simulink model "tutorial3"  (R2023b)
settings: Solver=FixedStepAuto  StartTime=0.0  StopTime=10.0  FixedStep=1e-3  RelTol=1e-3  EnableMultiTasking=on
libraries: frdmk64flib x5, etargetslib x2
settings Model: ExtModeTrigDuration=5  Creator=user  LastModifiedBy=user
settings OptimizationCC: EnhancedBackFolding=on  PassReuseOutputArgsAs=Individual arguments  ZeroExternalMemoryAtStartup=off  ZeroInternalMemoryAtStartup=off  MaxStackSize=64  OptimizeBlockOrder=speed  DifferentSizesBufferReuse=on  OptimizationCustomize=off  EfficientTunableParamExpr=on
settings DebuggingCC: ParameterTunabilityLossMsg=error
settings HardwareCC: ProdBitPerPointer=32  ProdBitPerSizeT=32  ProdBitPerPtrDiffT=32  ProdLargestAtomicInteger=Long  ProdLargestAtomicFloat=Double  ProdWordSize=32  ProdHWDeviceType=ARM Compatible->ARM Cortex
settings SFSimCC: MATLABDynamicMemAlloc=off
settings RTWCC: Description=Embedded Coder  SystemTargetFile=ert.tlc  HardwareBoard=NXP FRDM-K64F  TLCOptions="-aInlineSetEventsForThisBaseRateFcn=TLC_FALSE -aSuppressMultiTaskScheduler=TLC_FALSE  -aRateBasedStepFcn=0"  TemplateMakefile=ert_default_tmf  Toolchain=GNU Tools for ARM Embedded Processors
settings CodeAppCC: ForceParamTrailComments=on  IgnoreCustomStorageClasses=off  OperatorAnnotations=on  SimulinkDataObjDesc=on  SFDataObjDesc=on  InsertBlockDesc=on
settings ERTTargetCC: ExtModeTransport=4  ExtModeMexFile=sendToCommService

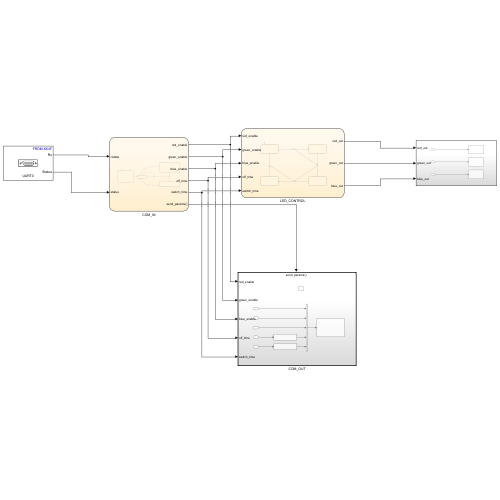
[thumbnail: Simulink's stored preview of the top-level diagram]
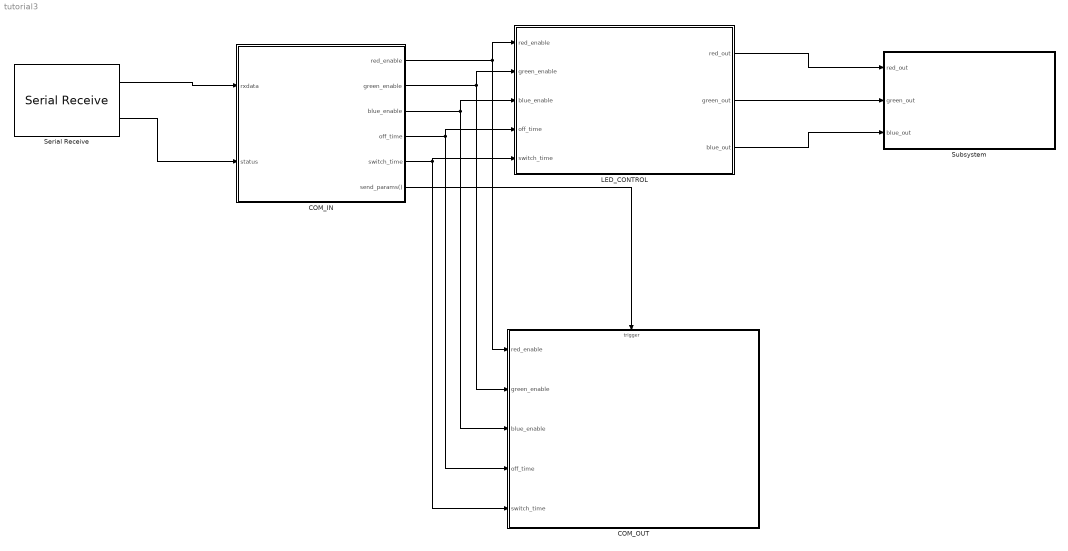
== system tutorial3 ==
  COM_IN : Stateflow chart  TreatAsAtomicUnit=on
  COM_OUT : Subsystem  TreatAsAtomicUnit=on
  LED_CONTROL : Stateflow chart  TreatAsAtomicUnit=on
  Serial Receive : frdmk64flib/Serial Receive  SCIModule=0  Baudrate=uint32(9600)  Parity=None  StopBits=1  HardwareFlowControl=None  ByteOrder=LittleEndian  DataType=uint8  DataLength=10  BlockingMode=off  OutputStatus=on  SampleTime=-1
  Subsystem : Subsystem
  wires:
  Serial Receive/1 -> COM_IN/1(rxdata)
  Serial Receive/2 -> COM_IN/2(status)
  COM_IN/1(red_enable) -> COM_OUT/1(red_enable), LED_CONTROL/1(red_enable)
  COM_IN/2(green_enable) -> COM_OUT/2(green_enable), LED_CONTROL/2(green_enable)
  COM_IN/3(blue_enable) -> COM_OUT/3(blue_enable), LED_CONTROL/3(blue_enable)
  COM_IN/4(off_time) -> COM_OUT/4(off_time), LED_CONTROL/4(off_time)
  COM_IN/5(switch_time) -> COM_OUT/5(switch_time), LED_CONTROL/5(switch_time)
  LED_CONTROL/1(red_out) -> Subsystem/1(red_out)
  LED_CONTROL/2(green_out) -> Subsystem/2(green_out)
  LED_CONTROL/3(blue_out) -> Subsystem/3(blue_out)
  COM_IN/6(send_params()) -> COM_OUT/Trigger

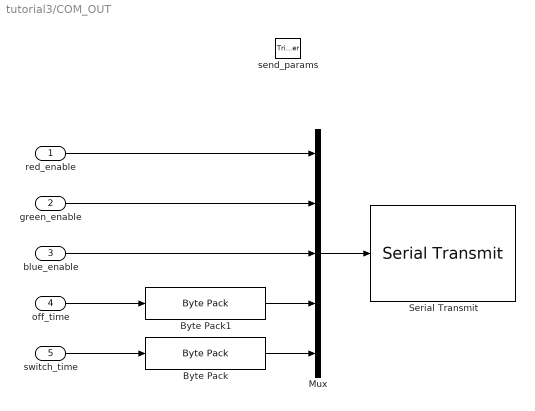
== system tutorial3/COM_OUT ==
  red_enable : Inport  OutDataTypeStr=uint8
  green_enable : Inport  Port=2  OutDataTypeStr=uint8
  blue_enable : Inport  Port=3  OutDataTypeStr=uint8
  off_time : Inport  Port=4  OutDataTypeStr=single
  switch_time : Inport  Port=5  OutDataTypeStr=uint16
  send_params : TriggerPort  TriggerType=function-call  VariantControl=(inherit)
  Byte Pack : etargetslib/Byte Pack  datatypes={'single'}  byteAlign=1
  Byte Pack1 : etargetslib/Byte Pack  datatypes={'single'}  byteAlign=1
  Mux : Mux  Inputs=5
  Serial Transmit : frdmk64flib/Serial Transmit  SCIModule=0  Baudrate=uint32(9600)  Parity=None  StopBits=1  HardwareFlowControl=None  ByteOrder=LittleEndian  BlockingMode=on  OutputStatus=off
  wires:
  Byte Pack/1 -> Mux/5
  off_time/1 -> Byte Pack1/1
  blue_enable/1 -> Mux/3
  switch_time/1 -> Byte Pack/1
  green_enable/1 -> Mux/2
  Byte Pack1/1 -> Mux/4
  red_enable/1 -> Mux/1
  Mux/1 -> Serial Transmit/1

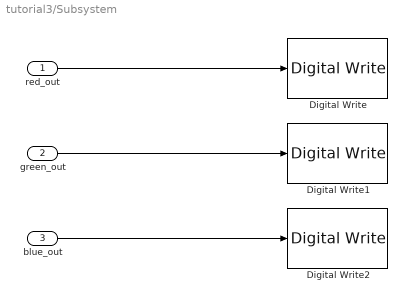
== system tutorial3/Subsystem ==
  red_out : Inport  OutDataTypeStr=boolean
  green_out : Inport  Port=2  OutDataTypeStr=boolean
  blue_out : Inport  Port=3  OutDataTypeStr=boolean
  Digital Write : frdmk64flib/Digital Write  Whichpin=RED_LED
  Digital Write1 : frdmk64flib/Digital Write  Whichpin=GREEN_LED
  Digital Write2 : frdmk64flib/Digital Write  Whichpin=BLUE_LED
  wires:
  red_out/1 -> Digital Write/1
  green_out/1 -> Digital Write1/1
  blue_out/1 -> Digital Write2/1

== stateflow chart tutorial3/LED_CONTROL ==
  state OFF
    entry:
    red_out = 0;
    green_out = 0;
    blue_out = 0;
  state RED_ON
    entry:
    red_out = 1;
    green_out = 0;
    blue_out = 0;
  state BLUE_ON
    entry:
    red_out = 0;
    green_out = 0;
    blue_out = 1;
  state GREEN_ON
    entry:
    red_out = 0;
    green_out = 1;
    blue_out = 0;
  (default) -> OFF
  OFF -> (junction 6) : [after(off_time, sec)]
  (junction 6) -> RED_ON [order 1] : [red_enable == 1]
  (junction 6) -> (junction 8) [order 2]
  (junction 7) -> OFF
  RED_ON -> (junction 8) : [after(switch_time, msec)]
  (junction 9) -> (junction 7) [order 2]
  (junction 8) -> (junction 9) [order 2]
  BLUE_ON -> (junction 7) : [after(switch_time, msec)]
  (junction 8) -> GREEN_ON [order 1] : [green_enable == 1]
  (junction 9) -> BLUE_ON [order 1] : [blue_enable == 1]
  GREEN_ON -> (junction 9) : [after(switch_time, msec)]
  data: red_out output boolean; green_out output boolean; red_enable input uint8; green_enable input uint8; blue_enable input uint8; off_time input single; switch_time input uint16; blue_out output boolean

== stateflow chart tutorial3/COM_IN ==
  state SET_PARAM
    entry:
    red_enable = rxdata(3);
    green_enable = rxdata(4);
    blue_enable = rxdata(5);
    off_time = typecast(rxdata(6:9), 'single');
    switch_time = typecast(rxdata(10:11), 'unit16');
  state INITIAL
    % Set the initial values of parameters
    entry:
    red_enable = 1;
    green_enable = 1;
    blue_enable = 1;
    off_time = 0.5; % In Seconds
    switch_time = 200; % In Milliseconds
  state STANDBY
    % Waiting for COM
  state ECHO_PARAM
    entry:
    send_params();
  SET_PARAM -> STANDBY
  (default) -> INITIAL
  (junction 9) -> STANDBY [order 2]
  (junction 11) -> SET_PARAM [order 1] : [rxdata(2) == hex2dec('55')]
  INITIAL -> STANDBY
  STANDBY -> (junction 9) : [status == 0]
  (junction 9) -> (junction 11) [order 1] : [rxdata(1) == hex2dec('16')]
  (junction 11) -> ECHO_PARAM [order 2] : [rxdata(2) == hex2dec('22')]
  ECHO_PARAM -> STANDBY
  data: red_enable output unit8; rxdata input uint8; green_enable output uint8; blue_enable output unit8; off_time output single; status input unit8; switch_time output uint16
  events: send_params output FUNCTION_CALL_EVENT
